simulink model "Demo3_model2"  (R2025b)
settings: Solver=VariableStepAuto  StartTime=0.0  StopTime=10.0  RelTol=1e-3
settings Model: Creator=FilipBabiec  LastModifiedBy=FilipBabiec

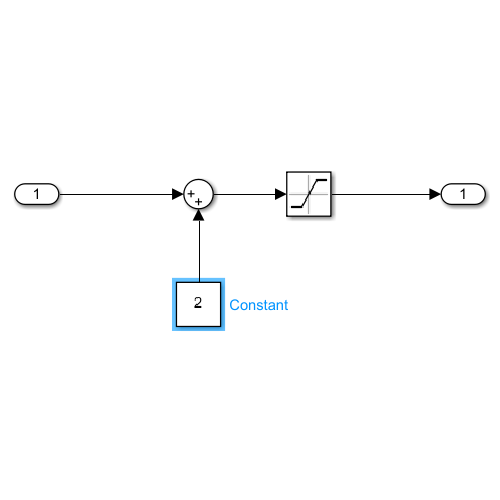
[thumbnail: Simulink's stored preview of the top-level diagram]
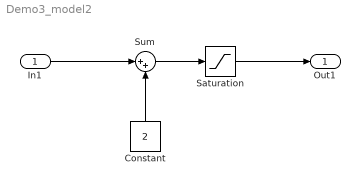
== system Demo3_model2 ==
  In1 : Inport
  Constant : Constant  Value=2
  Saturation : Saturate
  Sum : Sum  Inputs=|++
  Out1 : Outport
  wires:
  In1/1 -> Sum/1
  Constant/1 -> Sum/2
  Sum/1 -> Saturation/1
  Saturation/1 -> Out1/1
